simulink subsystem "RefMdl"  (R2021b)
settings: Solver=VariableStepAuto  StartTime=0.0  StopTime=10.0  RelTol=1e-3
values from neighbouring files (symbols this model uses):
  PredictionHorizon = 30    [setupscript.m]
  Ts = 0.1    [setupscript.m]
libraries: mpcadaslib x1, trackingutilitieslib x1, drivinglib x1
settings Model: Creator=Milin  LastModifiedBy=Milin.Patel
settings SolverCC: AlgebraicLoopSolver=TrustRegion
settings DebuggingCC: SFMachineParentedDataDiag=warning

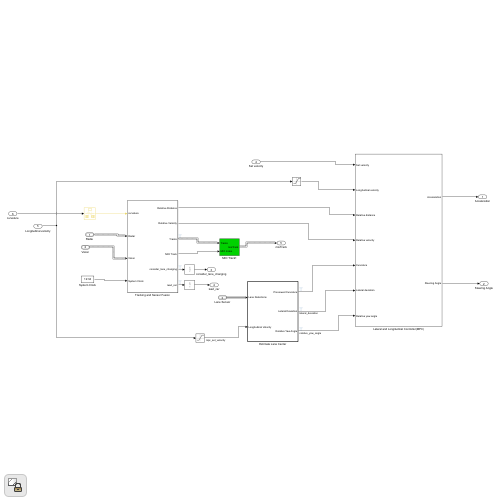
[thumbnail: Simulink's stored preview of the top-level diagram]
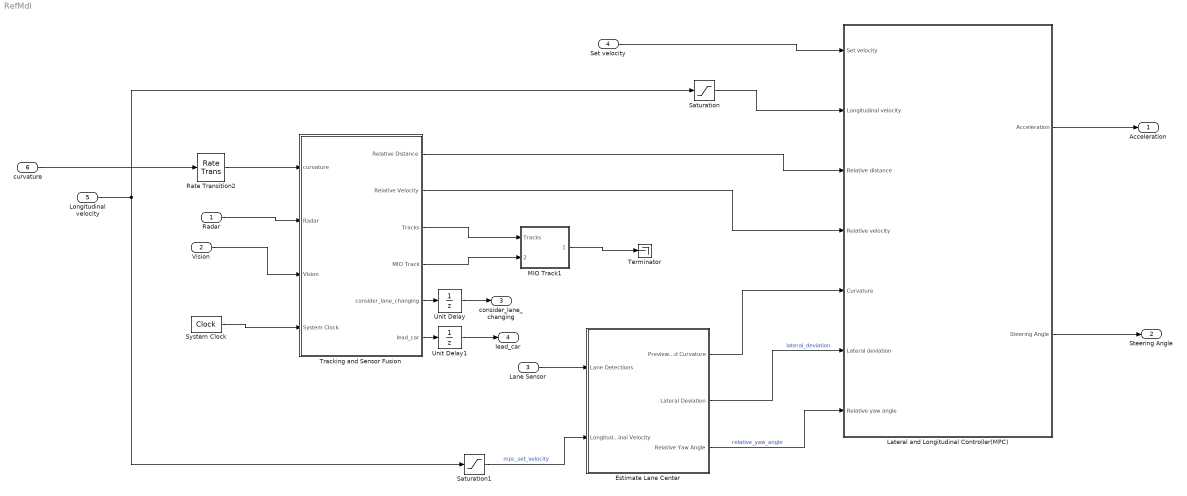
== system RefMdl ==
  Radar : Inport  OutDataTypeStr=Bus: BusRadar  PortDimensions=[1 1]  BusOutputAsStruct=on
  Vision : Inport  Port=2  OutDataTypeStr=Bus: BusVision  PortDimensions=[1 1]  BusOutputAsStruct=on
  Lane Sensor : Inport  Port=3  OutDataTypeStr=Bus: LaneSensor  PortDimensions=[1 1]
  Set velocity : Inport  Port=4
  Longitudinal velocity : Inport  Port=5
  curvature : Inport  Port=6  PortDimensions=[1 1]  SampleTime=[0.10000000000000001,0]
  Estimate Lane Center : Subsystem  TreatAsAtomicUnit=on  VariantControl=v2
      settings: RTWFileNameOpts=Use function name
  Lateral and Longitudinal Controller(MPC) : Subsystem
  MIO Track1 : Subsystem
  Rate Transition2 : RateTransition  OutPortSampleTime=Ts
  Saturation : Saturate  UpperLimit=100  LowerLimit=0.00001
  Saturation1 : Saturate  UpperLimit=inf  LowerLimit=0.0001
  System Clock : DigitalClock  SampleTime=Ts
  Terminator : Terminator
  Tracking and Sensor Fusion : Subsystem
  Unit Delay : UnitDelay  SampleTime=-1  HasFrameUpgradeWarning=on
  Unit Delay1 : UnitDelay  SampleTime=-1  HasFrameUpgradeWarning=on
  Acceleration : Outport  Unit=m/s^2
  Steering Angle : Outport  Port=2  Unit=rad
  consider_lane_changing : Outport  Port=3
  lead_car : Outport  Port=4
  wires:
  Lateral and Longitudinal Controller(MPC)/1(Acceleration) -> Acceleration/1
  Lateral and Longitudinal Controller(MPC)/2(Steering Angle) -> Steering Angle/1
  Lane Sensor/1 -> Estimate Lane Center/1(Lane Detections)
  Set velocity/1 -> Lateral and Longitudinal Controller(MPC)/1(Set velocity)
  Longitudinal velocity/1 -> Saturation1/1, Saturation/1
  Saturation/1 -> Lateral and Longitudinal Controller(MPC)/2(Longitudinal velocity)
  Tracking and Sensor Fusion/1(Relative Distance) -> Lateral and Longitudinal Controller(MPC)/3(Relative distance)
  Tracking and Sensor Fusion/2(Relative Velocity) -> Lateral and Longitudinal Controller(MPC)/4(Relative velocity)
  Tracking and Sensor Fusion/3(Tracks) -> MIO Track1/1(Tracks)
  Tracking and Sensor Fusion/4(MIO Track) -> MIO Track1/2(MIO Index)
  Tracking and Sensor Fusion/5(consider_lane_changing) -> Unit Delay/1
  Unit Delay/1 -> consider_lane_changing/1
  Tracking and Sensor Fusion/6(lead_car) -> Unit Delay1/1
  Unit Delay1/1 -> lead_car/1
  System Clock/1 -> Tracking and Sensor Fusion/4(System Clock)
  Radar/1 -> Tracking and Sensor Fusion/2(Radar)
  Vision/1 -> Tracking and Sensor Fusion/3(Vision)
  curvature/1 -> Rate Transition2/1
  Estimate Lane Center/1(Previewed Curvature) -> Lateral and Longitudinal Controller(MPC)/5(Curvature)
  Estimate Lane Center/2(Lateral Deviation) -> Lateral and Longitudinal Controller(MPC)/6(Lateral deviation)  "lateral_deviation"
  Estimate Lane Center/3(Relative Yaw Angle) -> Lateral and Longitudinal Controller(MPC)/7(Relative yaw angle)  "relative_yaw_angle"
  Saturation1/1 -> Estimate Lane Center/2(Longitudinal Velocity)  "mpc_set_velocity"
  Rate Transition2/1 -> Tracking and Sensor Fusion/1(curvature)
  MIO Track1/1(mioTrack) -> Terminator/1

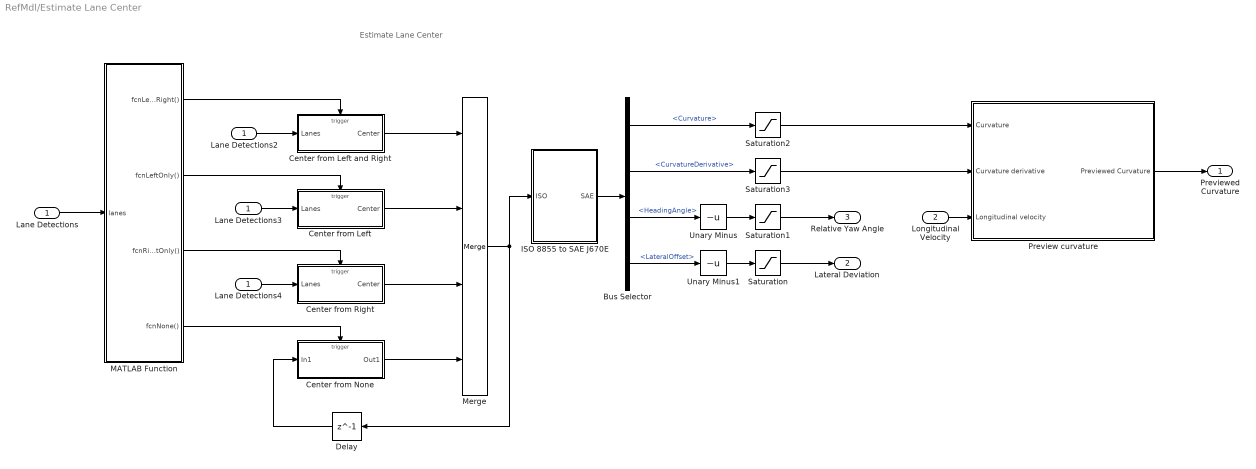
== system RefMdl/Estimate Lane Center ==
  note: Estimate Lane Center
  Lane Detections : Inport
  Longitudinal Velocity : Inport  Port=2
  Bus Selector : BusSelector  OutputSignals=Curvature,CurvatureDerivative,HeadingAngle,LateralOffset
  Center from Left : Subsystem  TreatAsAtomicUnit=on
  Center from Left and Right : Subsystem  TreatAsAtomicUnit=on
  Center from None : Subsystem  TreatAsAtomicUnit=on
  Center from Right : Subsystem  TreatAsAtomicUnit=on
  Delay : Delay  DelayLength=1
  ISO 8855 to SAE J670E : Subsystem
  Lane Detections2 : InportShadow
  Lane Detections3 : InportShadow
  Lane Detections4 : InportShadow
  MATLAB Function : MATLAB Function  TreatAsAtomicUnit=on
  Merge : Merge  Inputs=4
  Preview curvature : Subsystem
  Saturation : Saturate
  Saturation1 : Saturate  UpperLimit=0.6  LowerLimit=-0.6
  Saturation2 : Saturate  UpperLimit=0.15  LowerLimit=-0.15
  Saturation3 : Saturate  UpperLimit=0.06  LowerLimit=-0.06
  Unary Minus : UnaryMinus
  Unary Minus1 : UnaryMinus
  Previewed Curvature : Outport  VectorParamsAs1DForOutWhenUnconnected=off
  Lateral Deviation : Outport  Port=2  VectorParamsAs1DForOutWhenUnconnected=off
  Relative Yaw Angle : Outport  Port=3  VectorParamsAs1DForOutWhenUnconnected=off
  wires:
  Center from Right/1(Center) -> Merge/3
  Lane Detections4/1 -> Center from Right/1(Lanes)
  Lane Detections/1 -> MATLAB Function/1(lanes)
  Lane Detections3/1 -> Center from Left/1(Lanes)
  MATLAB Function/1(fcnLeftAndRight()) -> Center from Left and Right/Trigger
  MATLAB Function/4(fcnNone()) -> Center from None/Trigger
  Lane Detections2/1 -> Center from Left and Right/1(Lanes)
  Saturation3/1 -> Preview curvature/2(Curvature derivative)
  Center from Left and Right/1(Center) -> Merge/1
  Center from None/1(Out1) -> Merge/4
  MATLAB Function/3(fcnRightOnly()) -> Center from Right/Trigger
  MATLAB Function/2(fcnLeftOnly()) -> Center from Left/Trigger
  Unary Minus/1 -> Saturation1/1
  Bus Selector/4 -> Unary Minus1/1  "<LateralOffset>"
  Unary Minus1/1 -> Saturation/1
  Center from Left/1(Center) -> Merge/2
  Saturation2/1 -> Preview curvature/1(Curvature)
  Merge/1 -> Delay/1, ISO 8855 to SAE J670E/1(ISO)
  Bus Selector/2 -> Saturation3/1  "<CurvatureDerivative>"
  Bus Selector/1 -> Saturation2/1  "<Curvature>"
  Bus Selector/3 -> Unary Minus/1  "<HeadingAngle>"
  Saturation1/1 -> Relative Yaw Angle/1
  Longitudinal Velocity/1 -> Preview curvature/3(Longitudinal velocity)
  Saturation/1 -> Lateral Deviation/1
  ISO 8855 to SAE J670E/1(SAE) -> Bus Selector/1
  Delay/1 -> Center from None/1(In1)
  Preview curvature/1(Previewed Curvature) -> Previewed Curvature/1

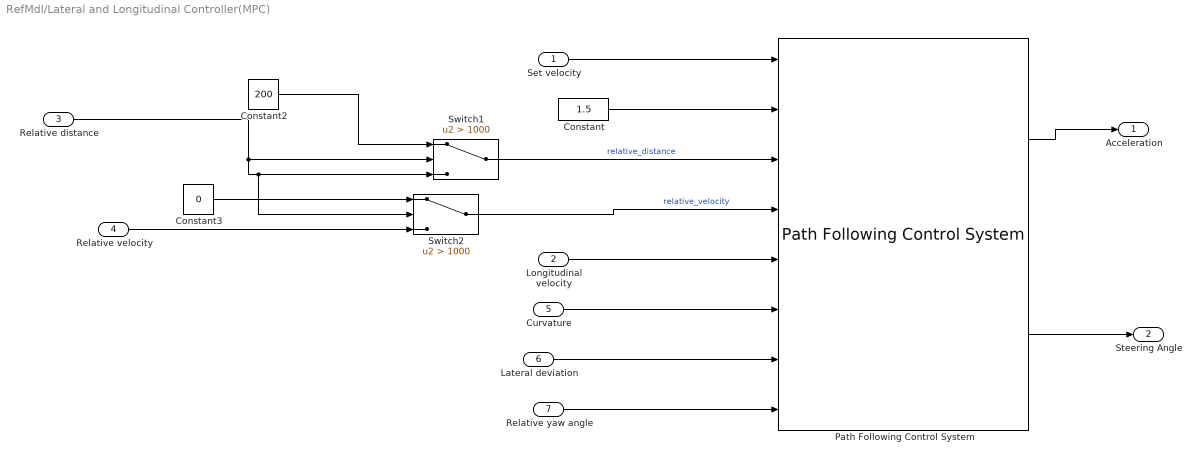
== system RefMdl/Lateral and Longitudinal Controller(MPC) ==
  Set velocity : Inport
  Longitudinal velocity : Inport  Port=2
  Relative distance : Inport  Port=3
  Relative velocity : Inport  Port=4
  Curvature : Inport  Port=5
  Lateral deviation : Inport  Port=6
  Relative yaw angle : Inport  Port=7
  Constant : Constant  Value=1.5
  Constant2 : Constant  Value=200
  Constant3 : Constant  Value=0
  Path Following Control System : mpcadaslib/Path Following Control System  VariantControl=Variant2  ModelType=Use vehicle parameters  VehicleMass=1575  VehicleYawInertia=2875  LengthToFront=1.2  LengthToRear=1.6  FrontTireStiffness=19000  RearTireStiffness=33000  AccelTimeConstant=0.5  EgoModelMatrixA=[-2,zeros(1,3);1,zeros(1,3);zeros(1,2),-4.4021,-12.4603;zeros(1,2),1.3913,-5.1868]  EgoModelMatrixB=[2,zeros(1,3);zeros(1,2),24.1270,15.8609]'  EgoModelMatrixC=[zeros(3,1),eye(3)]  InitialLongVel=v0_ego  TransportLag=Ts  spaceCtrl=on  DefaultSpacing=default_spacing  MinSteering=min_steer  umin_ext=off  MaxSteering=max_steer  umax_ext=off  MinAcceleration=min_ac  amin_ext=off  MaxAcceleration=max_ac  amax_ext=off  Ts=Ts  PredictionHorizon=30  ControlHorizon=2  LongWeight=0.1  LateralWeight=1  AccelRateWeight=0.1  SteerRateWeight=0.1  suboptimal=off  maxiter=10  datatypeopt=double  optmode=off  trackmode=off
      settings: SourceProductBaseCode=MP
  Switch1 : Switch  Criteria=u2 > Threshold  Threshold=1000
  Switch2 : Switch  Criteria=u2 > Threshold  Threshold=1000
  Acceleration : Outport
  Steering Angle : Outport  Port=2
  wires:
  Switch2/1 -> Path Following Control System/4  "relative_velocity"
  Switch1/1 -> Path Following Control System/3  "relative_distance"
  Relative velocity/1 -> Switch2/3
  Relative distance/1 -> Switch1/2, Switch1/3, Switch2/2
  Constant2/1 -> Switch1/1
  Constant3/1 -> Switch2/1
  Constant/1 -> Path Following Control System/2
  Relative yaw angle/1 -> Path Following Control System/8
  Path Following Control System/1 -> Acceleration/1
  Set velocity/1 -> Path Following Control System/1
  Lateral deviation/1 -> Path Following Control System/7
  Curvature/1 -> Path Following Control System/6
  Longitudinal velocity/1 -> Path Following Control System/5
  Path Following Control System/2 -> Steering Angle/1

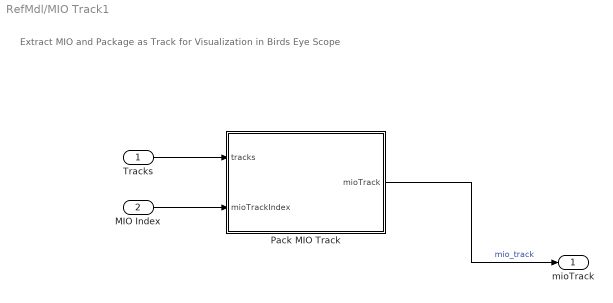
== system RefMdl/MIO Track1 ==
  note: Extract MIO and Package as Track for Visualization in Birds Eye Scope
  Tracks : Inport
  MIO Index : Inport  Port=2
  Pack MIO Track : MATLAB Function  TreatAsAtomicUnit=on
  mioTrack : Outport
  wires:
  MIO Index/1 -> Pack MIO Track/2(mioTrackIndex)
  Tracks/1 -> Pack MIO Track/1(tracks)
  Pack MIO Track/1(mioTrack) -> mioTrack/1  "mio_track"

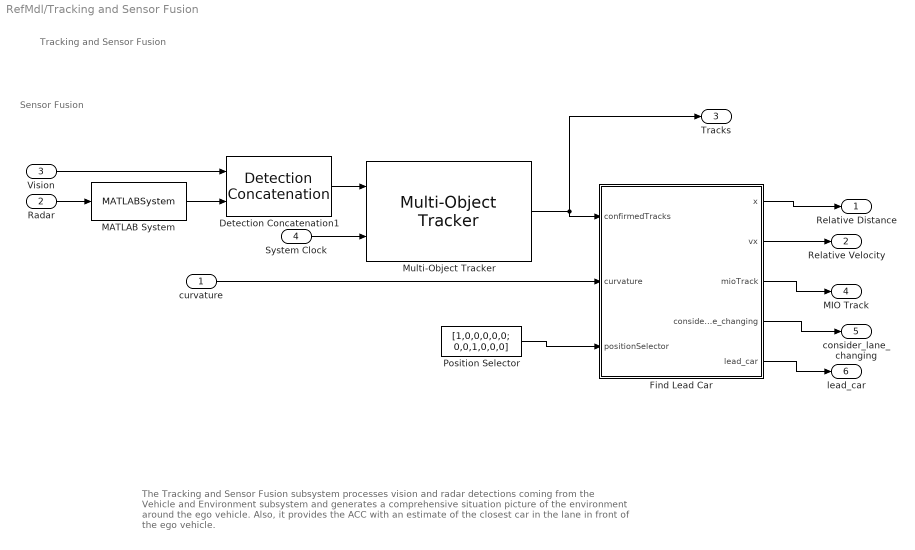
== system RefMdl/Tracking and Sensor Fusion ==
  note: The Tracking and Sensor Fusion subsystem processes vision and radar
      | detections coming from the Vehicle and Environment subsystem and
      | generates a comprehensive situation picture of the environment around
      | the ego vehicle. Also, it provides the ACC with an estimate of the closest
      | car in the lane in front of the ego vehicle.
  note: Tracking and Sensor Fusion
  note: Sensor Fusion
  curvature : Inport  PortDimensions=[1 1]  SampleTime=[0.10000000000000001,0]  BusOutputAsStruct=on
  Radar : Inport  Port=2  OutDataTypeStr=Bus: BusRadar  PortDimensions=[1 1]  BusOutputAsStruct=on
  Vision : Inport  Port=3  OutDataTypeStr=Bus: BusVision  PortDimensions=[1 1]  BusOutputAsStruct=on
  System Clock : Inport  Port=4  OutDataTypeStr=double  PortDimensions=[1 1]  SampleTime=[0.10000000000000001,0]
  Detection Concatenation1 : trackingutilitieslib/Detection Concatenation  NumInputs=2  BusNameSource=Auto  BusName=BusDetectionConcatenation1  SimulateUsing=Interpreted execution
      settings: SourceProductBaseCode=AE,DR,TF,RA,UV,VE
  Find Lead Car : MATLAB Function  TreatAsAtomicUnit=on
  MATLAB System : MATLABSystem  System=helperClusterDetections  ClusterSize=4  BusNameSource=Auto  BusName=BusClusterDetections  SimulateUsing=Interpreted execution
      mask Type: helperClusterDetections
      mask Display:
      | disp(['Detection' char(10) 'Clustering']);
      | port_label('input',1,'In');
      | port_label('output',1,'Out');
  Multi-Object Tracker : drivinglib/Multi-Object Tracker  TrackerIndex=uint32( 0 )  FilterInitializationFcn=initcvekf  AssignmentThreshold=20  ConfirmationThreshold=[ 2, 3 ]  DeletionThreshold=[ 5, 5 ]  MaxNumTracks=20  MaxNumSensors=2  OOSMHandling=Terminate  StateParametersSimulink=struct  HasStateParametersInput=off  TimeInputSource=Input port  HasCostMatrixInput=off  HasDetectableTrackIDsInput=off  BusNameSource=Property  BusName=BusMultiObjectTracker1  TentativeTracksOutputPort=off  AllTracksOutputPort=off  SimulateUsing=Interpreted execution
      settings: SourceProductBaseCode=DR
  Position Selector : Constant  Value=[1,0,0,0,0,0; 0,0,1,0,0,0]
  Relative Distance : Outport  VectorParamsAs1DForOutWhenUnconnected=off
  Relative Velocity : Outport  Port=2  VectorParamsAs1DForOutWhenUnconnected=off
  Tracks : Outport  Port=3  OutDataTypeStr=Bus:BusMultiObjectTracker1  PortDimensions=[1 1]  SampleTime=[0.10000000000000001,0]  VectorParamsAs1DForOutWhenUnconnected=off  BusOutputAsStruct=on
  MIO Track : Outport  Port=4
  consider_lane_changing : Outport  Port=5
  lead_car : Outport  Port=6
  wires:
  curvature/1 -> Find Lead Car/2(curvature)
  Radar/1 -> MATLAB System/1
  Detection Concatenation1/1 -> Multi-Object Tracker/1
  Vision/1 -> Detection Concatenation1/1
  Multi-Object Tracker/1 -> Tracks/1, Find Lead Car/1(confirmedTracks)
  System Clock/1 -> Multi-Object Tracker/2
  MATLAB System/1 -> Detection Concatenation1/2
  Find Lead Car/3(mioTrack) -> MIO Track/1
  Find Lead Car/5(lead_car) -> lead_car/1
  Find Lead Car/4(consider_lane_changing) -> consider_lane_changing/1
  Find Lead Car/1(x) -> Relative Distance/1
  Position Selector/1 -> Find Lead Car/3(positionSelector)
  Find Lead Car/2(vx) -> Relative Velocity/1

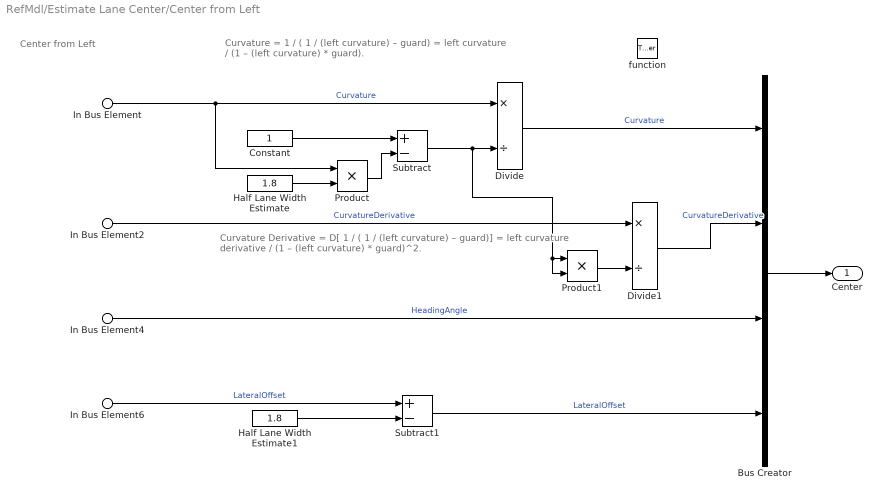
== system RefMdl/Estimate Lane Center/Center from Left ==
  note: Curvature
      | = 1 / ( 1 / (left curvature) – guard)
      | = left curvature / (1 – (left curvature) * guard).
  note: Center from Left
  note: Curvature Derivative
      | = D[ 1 / ( 1 / (left curvature) – guard)]
      | = left curvature derivative / (1 – (left curvature) * guard)^2.
  In Bus Element : Inport  PortName=Lanes  Element=Left.Curvature
  In Bus Element2 : Inport  PortName=Lanes  Element=Left.CurvatureDerivative
  In Bus Element4 : Inport  PortName=Lanes  Element=Left.HeadingAngle
  In Bus Element6 : Inport  PortName=Lanes  Element=Left.LateralOffset
  function : TriggerPort  TriggerType=function-call  VariantControl=Variant
  Bus Creator : BusCreator  Inputs=4
  Constant : Constant  OutDataTypeStr=Inherit: Inherit via back propagation
  Divide : Product  Inputs=*/
  Divide1 : Product  Inputs=*/
  Half Lane Width Estimate : Constant  Value=1.8  OutDataTypeStr=Inherit: Inherit via back propagation
  Half Lane Width Estimate1 : Constant  Value=1.8  OutDataTypeStr=Inherit: Inherit via back propagation
  Product : Product
  Product1 : Product
  Subtract : Sum  Inputs=+-
  Subtract1 : Sum  Inputs=+-
  Center : Outport  VectorParamsAs1DForOutWhenUnconnected=off
  wires:
  Bus Creator/1 -> Center/1
  Divide1/1 -> Bus Creator/2  "CurvatureDerivative"
  Divide/1 -> Bus Creator/1  "Curvature"
  In Bus Element4/1 -> Bus Creator/3  "HeadingAngle"
  Subtract1/1 -> Bus Creator/4  "LateralOffset"
  In Bus Element/1 -> Product/1, Divide/1  "Curvature"
  Subtract/1 -> Product1/2, Product1/1, Divide/2
  Half Lane Width Estimate/1 -> Product/2
  Constant/1 -> Subtract/1
  In Bus Element2/1 -> Divide1/1  "CurvatureDerivative"
  Product1/1 -> Divide1/2
  In Bus Element6/1 -> Subtract1/1  "LateralOffset"
  Half Lane Width Estimate1/1 -> Subtract1/2
  Product/1 -> Subtract/2

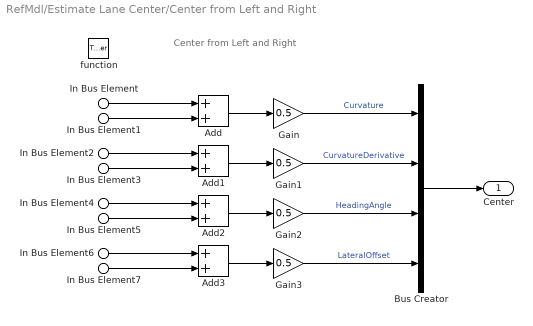
== system RefMdl/Estimate Lane Center/Center from Left and Right ==
  note: Center from Left and Right
  In Bus Element : Inport  PortName=Lanes  Element=Left.Curvature
  In Bus Element2 : Inport  PortName=Lanes  Element=Left.CurvatureDerivative
  In Bus Element4 : Inport  PortName=Lanes  Element=Left.HeadingAngle
  In Bus Element6 : Inport  PortName=Lanes  Element=Left.LateralOffset
  In Bus Element1 : Inport  PortName=Lanes  Element=Right.Curvature
  In Bus Element3 : Inport  PortName=Lanes  Element=Right.CurvatureDerivative
  In Bus Element5 : Inport  PortName=Lanes  Element=Right.HeadingAngle
  In Bus Element7 : Inport  PortName=Lanes  Element=Right.LateralOffset
  function : TriggerPort  TriggerType=function-call  VariantControl=Variant
  Add{,1..3} (4 alike) : Sum
  Bus Creator : BusCreator  Inputs=4
  Gain{,1..3} (4 alike) : Gain  Gain=0.5
  Center : Outport  VectorParamsAs1DForOutWhenUnconnected=off
  wires:
  Add/1 -> Gain/1
  Gain/1 -> Bus Creator/1  "Curvature"
  Add1/1 -> Gain1/1
  Gain1/1 -> Bus Creator/2  "CurvatureDerivative"
  Add2/1 -> Gain2/1
  Gain2/1 -> Bus Creator/3  "HeadingAngle"
  Add3/1 -> Gain3/1
  Gain3/1 -> Bus Creator/4  "LateralOffset"
  Bus Creator/1 -> Center/1
  In Bus Element/1 -> Add/1
  In Bus Element1/1 -> Add/2
  In Bus Element2/1 -> Add1/1
  In Bus Element3/1 -> Add1/2
  In Bus Element4/1 -> Add2/1
  In Bus Element5/1 -> Add2/2
  In Bus Element7/1 -> Add3/2
  In Bus Element6/1 -> Add3/1

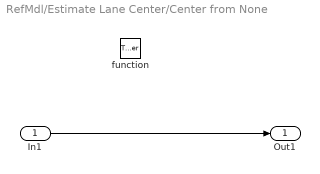
== system RefMdl/Estimate Lane Center/Center from None ==
  In1 : Inport
  function : TriggerPort  TriggerType=function-call  VariantControl=Variant
  Out1 : Outport  VectorParamsAs1DForOutWhenUnconnected=off
  wires:
  In1/1 -> Out1/1

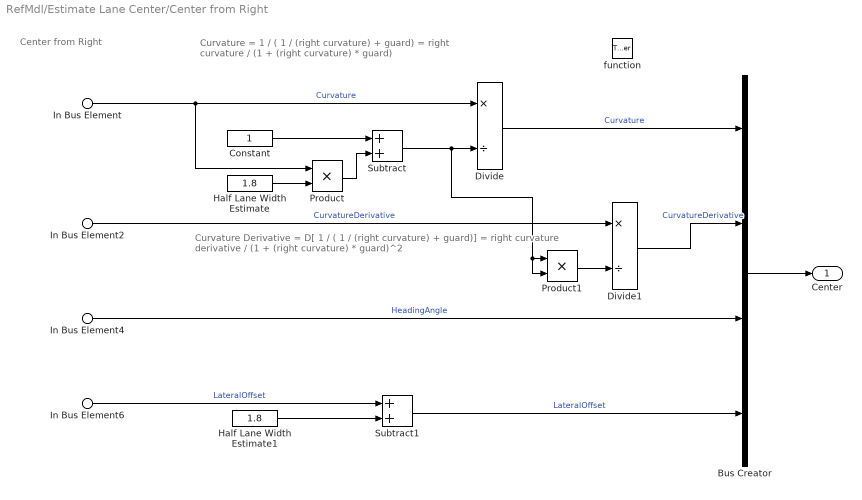
== system RefMdl/Estimate Lane Center/Center from Right ==
  note: Center from Right
  note: Curvature
      | = 1 / ( 1 / (right curvature) + guard)
      | = right curvature / (1 + (right curvature) * guard)
  note: Curvature Derivative
      | = D[ 1 / ( 1 / (right curvature) + guard)]
      | = right curvature derivative / (1 + (right curvature) * guard)^2
  In Bus Element : Inport  PortName=Lanes  Element=Right.Curvature
  In Bus Element2 : Inport  PortName=Lanes  Element=Right.CurvatureDerivative
  In Bus Element4 : Inport  PortName=Lanes  Element=Right.HeadingAngle
  In Bus Element6 : Inport  PortName=Lanes  Element=Right.LateralOffset
  function : TriggerPort  TriggerType=function-call  VariantControl=Variant
  Bus Creator : BusCreator  Inputs=4
  Constant : Constant  OutDataTypeStr=Inherit: Inherit via back propagation
  Divide : Product  Inputs=*/
  Divide1 : Product  Inputs=*/
  Half Lane Width Estimate : Constant  Value=1.8  OutDataTypeStr=Inherit: Inherit via back propagation
  Half Lane Width Estimate1 : Constant  Value=1.8  OutDataTypeStr=Inherit: Inherit via back propagation
  Product : Product
  Product1 : Product
  Subtract : Sum
  Subtract1 : Sum
  Center : Outport  VectorParamsAs1DForOutWhenUnconnected=off
  wires:
  In Bus Element2/1 -> Divide1/1  "CurvatureDerivative"
  Divide1/1 -> Bus Creator/2  "CurvatureDerivative"
  Product1/1 -> Divide1/2
  In Bus Element4/1 -> Bus Creator/3  "HeadingAngle"
  Half Lane Width Estimate1/1 -> Subtract1/2
  In Bus Element6/1 -> Subtract1/1  "LateralOffset"
  Divide/1 -> Bus Creator/1  "Curvature"
  Subtract1/1 -> Bus Creator/4  "LateralOffset"
  Bus Creator/1 -> Center/1
  In Bus Element/1 -> Product/1, Divide/1  "Curvature"
  Subtract/1 -> Product1/2, Product1/1, Divide/2
  Constant/1 -> Subtract/1
  Product/1 -> Subtract/2
  Half Lane Width Estimate/1 -> Product/2

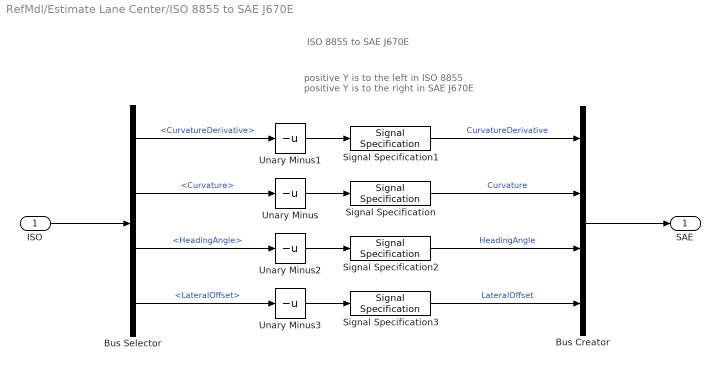
== system RefMdl/Estimate Lane Center/ISO 8855 to SAE J670E ==
  note: ISO 8855 to SAE J670E
  note: positive Y is to the left in ISO 8855
      | positive Y is to the right in SAE J670E
  ISO : Inport
  Bus Creator : BusCreator  Inputs=4
  Bus Selector : BusSelector  OutputSignals=CurvatureDerivative,Curvature,HeadingAngle,LateralOffset
  Signal Specification : SignalSpecification  Unit=1/m^2
  Signal Specification1 : SignalSpecification  Unit=1/m
  Signal Specification2 : SignalSpecification  Unit=rad
  Signal Specification3 : SignalSpecification  Unit=m
  Unary Minus{,1..3} (4 alike) : UnaryMinus
  SAE : Outport  VectorParamsAs1DForOutWhenUnconnected=off
  wires:
  Signal Specification3/1 -> Bus Creator/4  "LateralOffset"
  Signal Specification2/1 -> Bus Creator/3  "HeadingAngle"
  Signal Specification1/1 -> Bus Creator/1  "CurvatureDerivative"
  Unary Minus/1 -> Signal Specification/1
  Unary Minus3/1 -> Signal Specification3/1
  Unary Minus2/1 -> Signal Specification2/1
  Unary Minus1/1 -> Signal Specification1/1
  Signal Specification/1 -> Bus Creator/2  "Curvature"
  Bus Creator/1 -> SAE/1
  Bus Selector/4 -> Unary Minus3/1  "<LateralOffset>"
  Bus Selector/3 -> Unary Minus2/1  "<HeadingAngle>"
  Bus Selector/1 -> Unary Minus1/1  "<CurvatureDerivative>"
  Bus Selector/2 -> Unary Minus/1  "<Curvature>"
  ISO/1 -> Bus Selector/1

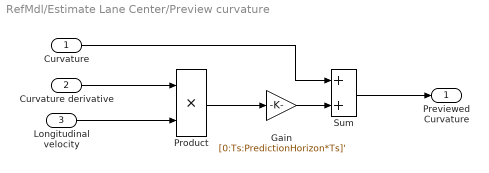
== system RefMdl/Estimate Lane Center/Preview curvature ==
  Curvature : Inport
  Curvature derivative : Inport  Port=2
  Longitudinal velocity : Inport  Port=3
  Gain : Gain  Gain=[0:Ts:PredictionHorizon*Ts]'
  Product : Product
  Sum : Sum
  Previewed Curvature : Outport  VectorParamsAs1DForOutWhenUnconnected=off
  wires:
  Curvature derivative/1 -> Product/1
  Longitudinal velocity/1 -> Product/2
  Product/1 -> Gain/1
  Gain/1 -> Sum/2
  Curvature/1 -> Sum/1
  Sum/1 -> Previewed Curvature/1

== matlab function RefMdl/Tracking and Sensor Fusion/Find Lead Car ==
  data: confirmedTracks input; x output size=[1 1]; vx output size=[1 1]; curvature input; mioTrack output; positionSelector input; consider_lane_changing output; lead_car output
function [x,vx,mioTrack,consider_lane_changing,lead_car] = findLeadCar(confirmedTracks,curvature, positionSelector)
% This function finds the lead car: a car in front of the ego car that
% satisfies all the criteria below:
% * Within the ego car's lane.
% * In front of the ego car.
% * Closest to the ego car.

% Note: If you change state definition, change the following:
%       State = [x;vx;y;vy;z;vz] (3D constant velocity)
numStates = 6;

% Initialize outputs and parameters
maxX = cast(1000, 'like', confirmedTracks.Tracks(1).State);  % Far enough forward so that no track is expected to exceed this distance
trackID = 0;

% If lane detection is not available, the ego car is assumed to be located
% in the middle of its lane. The lane width is assumed to be 3.6m, typical
% highway lane width.
laneWidth = 3.6;
halfLaneWidth = laneWidth/2;

% if lane.Left.Strength > 0.01
%     lb =  lane.Left.Curvature/2;                          
%lane.Left.CurvatureDerivative/6,...
% 
% %         lane.Left.HeadingAngle,...
% %         lane.Left.LateralOffset];
% else
%     lb = single([0,0,0,halfLaneWidth]);
% end
% 
% if lane.Right.Strength > 0.01
%     rb =  lane.Right.Curvature/2;
%     
% %     [lane.Right.CurvatureDerivative/6,...
% %         lane.Right.Curvature/2,...
% %         lane.Right.HeadingAngle,...
% %         lane.Right.LateralOffset];
% else
%     rb = single([0,0,0,-halfLaneWidth]);    
% end
% initialize MIOs
EgoFront = struct(...
    'TrackIndex', uint32(0),...
    'Position', double([0 0]'), ...
    'Velocity', double([0 0]'), ...
    'RangeMagnitude', double(2000), ...  % default range = big number (ex. 2000)
    'VelocityMagnitude', double(0), ...
    'TTC', double(100));

% EgoRear = struct(...
%     'TrackIndex', uint32(0),...
%     'Position', double([0 0]'), ...
%     'Velocity', double([0 0]'), ...
%     'RangeMagnitude', double(0), ...  
%     'VelocityMagnitude', double(0), ...
%     'TTC', double(0));



% LeftRear = struct(...
%     'TrackIndex', uint32(0),...
%     'Position', double([0 0]'), ...
%     'Velocity', double([0 0]'), ...
%     'RangeMagnitude', double(0), ...
%     'VelocityMagnitude', double(0), ...
%     'TTC', double(0));


% RightRear = struct(...
%     'TrackIndex', uint32(0),...
%     'Position', double([0 0]'), ...
%     'Velocity', double([0 0]'), ...
%     'RangeMagnitude', double(0), ...
%     'VelocityMagnitude', double(0), ...
%     'TTC', double(0));

%

for i = 1:confirmedTracks.NumTracks
    position = positionSelector * confirmedTracks.Tracks(i).State;
    x = position(1); % Longitudinal position of the track relative to ego
    y = position(2); % Lateral position of the track relative to ego
    
    

       yleftLane  = polyval([curvature/2, 0 , halfLaneWidth],x); % lateral position of left lane
        yrightLane = polyval([curvature/2, 0 ,-halfLaneWidth],x); % lateral position of right lane
        
     if x < maxX && x > 0 % No point checking otherwise
        % Find a new lead car
        if (yrightLane <= y) && (y <= yleftLane)
            maxX = x;
            trackID = i;
            EgoFront.TrackIndex = uint32(i);
        end
     end
    
end


if trackID>0
    mioState = confirmedTracks.Tracks(trackID).State;
    lead_car= 1;
else
    mioState = inf(numStates,1,'like',confirmedTracks.Tracks(1).State);
    lead_car = 0;
end

 
 

% Output:
x = mioState(1);    % Longitudinal position of the lead car
vx = mioState(2);   % Longitudinal velocity of the lead car
if confirmedTracks.NumTracks <=1 && abs(vx)<=1 && x>=18 && lead_car ==1
    % There is a front vehicle,the |relative velocity| is less than one,the 
    % relative distance is larger than 18,then consider to make lane change 
    % maneuver.
    consider_lane_changing = 1;
else
    consider_lane_changing = 0;
end
mioTrack = trackID; % Index of the most important track

end

== matlab function RefMdl/Estimate Lane Center/MATLAB Function ==
  data: lanes input
  events: fcnLeftAndRight output FUNCTION_CALL_EVENT; fcnLeftOnly output FUNCTION_CALL_EVENT; fcnRightOnly output FUNCTION_CALL_EVENT; fcnNone output FUNCTION_CALL_EVENT
function fcn(lanes)

leftStrength  = lanes.Left.Strength;
rightStrength = lanes.Right.Strength;

if (leftStrength > 0) && (rightStrength > 0)
   fcnLeftAndRight();
   
elseif leftStrength > 0
    fcnLeftOnly();
    
elseif rightStrength > 0
    fcnRightOnly();
    
else
    fcnNone();
end

== matlab function RefMdl/MIO Track1/Pack MIO Track ==
  data: tracks input; mioTrack output Bus: BusMultiObjectTracker1; mioTrackIndex input
function mioTrack = fcn(tracks, mioTrackIndex)
% Extract MIO track and package for visualization in Birds Eye Scope

mioTrack = tracks;

if mioTrackIndex > 0
    % First track represents MIO
    mioTrack.NumTracks = 1;
    mioTrack.Tracks(1) = tracks.Tracks(mioTrackIndex);
else
    % No valid MIO track
    mioTrack.NumTracks = 0;
end
